simulink model "dokladny_model"  (R2015a)
settings: Solver=ode45  StartTime=0.0  StopTime=czas_sym  MaxStep=tmax  RelTol=1e-3
values from neighbouring files (symbols this model uses):
  cpp = 1000    [z_identyfikacja.m]
  Cvg = cpw*row*Vg    (= 200400)    [z_identyfikacja.m]
  Cvs = cpb*rob*Vb    (= 56809984)    [z_identyfikacja.m]
  dFp = FpN*0.0    [dokladny.m]    (also in kupfmuller.m)
  dQg = QgN*0.1    [dokladny.m]    (also in kupfmuller.m; row_stanu.m; ss_tf.m; transmitancje.m = QgN*0.0)
  dTzew = 0    [dokladny.m]    (also in kupfmuller.m; row_stanu.m; ss_tf.m = 2; transmitancje.m = 2)
  Fp0 = wektor_Fp0(i)    [char_czestotliwosciowe.m]    (also in char_statyczne.m = [0 : FpN : (15*FpN)]; dokladny.m; kupfmuller.m; row_stanu.m)
  Kg = QgN/(TgN - TwewN)    (= 500)    [z_identyfikacja.m]
  Ks = Kw*a    (= 1241.66666667)    [z_identyfikacja.m]
  Kw = (QgN - cpp*rop*FpN*(TwewN - TzewN)) / (TwewN - TsN)    (= 827.777777778)    [z_identyfikacja.m]
  MTwew_dok = Kg + Kw    [dokladny.m]    (also in kupfmuller.m)
  Qg0 = wektor_Qg0(i)    [char_czestotliwosciowe.m]    (also in char_statyczne.m = [0.7*QgN : 0.1*QgN : (1.3*QgN)]; dokladny.m; kupfmuller.m; row_stanu.m)
  rop = 1.2    [z_identyfikacja.m]
  t0 = 40000    [dokladny.m]    (also in kupfmuller.m; row_stanu.m; transmitancje.m)
  Tg0 = -(Ks*MTw*Qg0 - Kw^2*Qg0 + Kw*MTw*Qg0 + P*Kg*Ks*Tzew0 + P*Kg*Kw*Tzew0 + Kg*Ks*Kw*Tzew0)/(Kg*(Kw^2 + Kg*Ks + Kg*Kw - Ks*MTw - Kw*MTw))    [dokladny.m]    (also in kupfmuller.m; row_stanu.m; ss_tf_support.m; transmitancje.m)
  Ts0 = -(Kw*Qg0 + P*Kw*Tzew0 - Kg*Ks*Tzew0 + Ks*MTw*Tzew0)/(Kw^2 + Kg*Ks + Kg*Kw - Ks*MTw - Kw*MTw)    [dokladny.m]    (also in kupfmuller.m; row_stanu.m; ss_tf_support.m; transmitancje.m)
  Tzew0 = wektor_Tzew0(i)    [char_czestotliwosciowe.m]    (also in char_statyczne.m = [0.7*TzewN : 0.1*TzewN : 1.3*TzewN]; dokladny.m; kupfmuller.m; row_stanu.m)
settings Model: Creator=Jacek  LastModifiedBy=Prezes
settings DataIOCC: LimitDataPoints=off

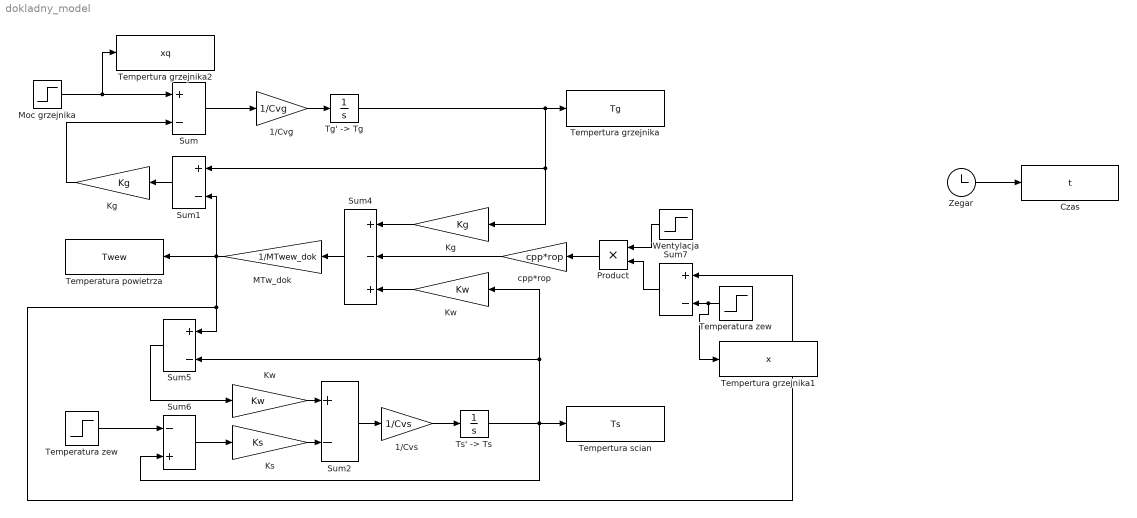
== system dokladny_model ==
  1/Cvg : Gain  Gain=1/Cvg
  1/Cvs : Gain  Gain=1/Cvs
  Czas : ToWorkspace  VariableName=t  SampleTime=-1
      settings: Save2DSignal=2-D array (concatenate along first dimension)
  Kg : Gain  Gain=Kg
  "Kg " : Gain  Gain=Kg
  Ks : Gain  Gain=Ks
  Kw : Gain  Gain=Kw
  "Kw " : Gain  Gain=Kw
  MTw_dok : Gain  Gain=1/MTwew_dok
  Moc grzejnika : Step  Time=t0  Before=Qg0  After=Qg0 + dQg  SampleTime=0
  Product : Product
  Sum{,1..2,5,7} (5 alike) : Sum  Inputs=+-
  Sum4 : Sum  Inputs=+-+
  Sum6 : Sum  Inputs=-+
  Temperatura powietrza : ToWorkspace  VariableName=Twew  SampleTime=-1
      settings: Save2DSignal=2-D array (concatenate along first dimension)
  Temperatura zew : Step  Time=t0  Before=Tzew0  After=Tzew0+ dTzew  SampleTime=0
  "Temperatura zew " : Step  Time=t0  Before=Tzew0  After=Tzew0+ dTzew  SampleTime=0
  Tempertura grzejnika : ToWorkspace  VariableName=Tg  SampleTime=-1
      settings: Save2DSignal=2-D array (concatenate along first dimension)
  Tempertura grzejnika1 : ToWorkspace  VariableName=x  SampleTime=-1
      settings: Save2DSignal=2-D array (concatenate along first dimension)
  Tempertura grzejnika2 : ToWorkspace  VariableName=xq  SampleTime=-1
      settings: Save2DSignal=2-D array (concatenate along first dimension)
  Tempertura scian : ToWorkspace  VariableName=Ts  SampleTime=-1
      settings: Save2DSignal=2-D array (concatenate along first dimension)
  "Tg' -> Tg" : Integrator  InitialCondition=Tg0
  "Ts' -> Ts" : Integrator  InitialCondition=Ts0
  Wentylacja : Step  Time=t0  Before=Fp0  After=Fp0+dFp  SampleTime=0
  Zegar : Clock
  cpp*rop : Gain  Gain=cpp*rop
  wires:
  Sum/1 -> 1/Cvg/1
  1/Cvg/1 -> "Tg' -> Tg"/1
  1/Cvs/1 -> "Ts' -> Ts"/1
  Sum2/1 -> 1/Cvs/1
  Kg/1 -> Sum/2
  Sum1/1 -> Kg/1
  Sum5/1 -> Kw/1
  Kw/1 -> Sum2/1
  Sum6/1 -> Ks/1
  Ks/1 -> Sum2/2
  Moc grzejnika/1 -> Tempertura grzejnika2/1, Sum/1
  Zegar/1 -> Czas/1
  Sum4/1 -> MTw_dok/1
  "Temperatura zew "/1 -> Sum6/1
  Temperatura zew/1 -> Tempertura grzejnika1/1, Sum7/2
  Wentylacja/1 -> Product/1
  Sum7/1 -> Product/2
  "Kw "/1 -> Sum4/3
  "Ts' -> Ts"/1 -> Sum6/2, Tempertura scian/1, Sum5/2, "Kw "/1
  cpp*rop/1 -> Sum4/2
  Product/1 -> cpp*rop/1
  "Kg "/1 -> Sum4/1
  "Tg' -> Tg"/1 -> Sum1/1, "Kg "/1, Tempertura grzejnika/1
  MTw_dok/1 -> Sum5/1, Sum7/1, Temperatura powietrza/1, Sum1/2
